simulink model "Quadcopter_LQG_Discrete"  (R2016b)
settings: Solver=ode45  StartTime=0.0  StopTime=33  RelTol=1e-3  EnableMultiTasking=on
undefined symbols (not defined in the file): A, B, C, D, F, kest, Ts, X0
settings Model: Creator=Toshiba  LastModifiedBy=AAstudillo
settings DataIOCC: LimitDataPoints=on  SaveFormat=Array  SignalLoggingSaveFormat=ModelDataLogs
settings OptimizationCC: LifeSpan=inf
settings DebuggingCC: SolverPrmCheckMsg=warning  MultiTaskDSMMsg=warning  MultiTaskCondExecSysMsg=none  SFUnexpectedBacktrackingDiag=warning  SFNoUnconditionalDefaultTransitionDiag=warning  SFExecutionAtInitializationDiag=none
settings HardwareCC: ProdBitPerPointer=32  ProdBitPerSizeT=32  ProdBitPerPtrDiffT=32  ProdLargestAtomicFloat=None  ProdIntDivRoundTo=Undefined  ProdEndianess=Unspecified  ProdWordSize=32  ProdHWDeviceType=32-bit Generic
settings ModelReferenceCC: PropagateSignalLabelsOutOfModel=off
settings GRTTargetCC: TargetLangStandard=C89/C90 (ANSI)  GeneratePreprocessorConditionals=Disable all
settings ConfigComp: CovMetricSettings=dw  CovHtmlReporting=on  CovSaveCumulativeToWorkspaceVar=on  CovSaveSingleToWorkspaceVar=on  CovExternalEMLEnable=off

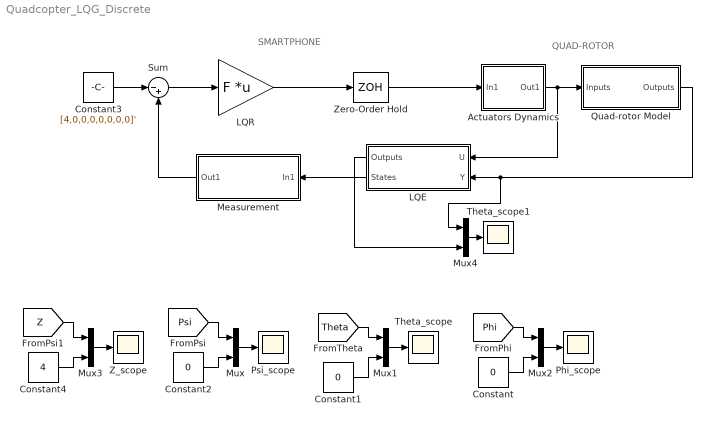
== system Quadcopter_LQG_Discrete ==
  note: QUAD-ROTOR
  note: SMARTPHONE
  Actuators Dynamics : Subsystem
  Constant : Constant  Value=0
  Constant1 : Constant  Value=0
  Constant2 : Constant  Value=0
  Constant3 : Constant  Value=[4,0,0,0,0,0,0,0]'
  Constant4 : Constant  Value=4
  LQE : Subsystem
  LQR : Gain  Gain=F  Multiplication=Matrix(K*u)
  Measurement : Subsystem
  Mux{,1..4} (5 alike) : Mux  Inputs=2
  Phi_scope : Scope
  Psi_scope : Scope
  Quad-rotor Model : Subsystem
  Sum : Sum  Inputs=|-+
  Theta_scope : Scope
  Theta_scope1 : Scope
  Z_scope : Scope
  Zero-Order Hold : ZeroOrderHold  SampleTime=Ts
  wires:
  Constant3/1 -> Sum/1
  Mux/1 -> Psi_scope/1
  Mux1/1 -> Theta_scope/1
  Mux2/1 -> Phi_scope/1
  [Psi] -> Mux/1
  Constant2/1 -> Mux/2
  [Theta] -> Mux1/1
  Constant1/1 -> Mux1/2
  [Phi] -> Mux2/1
  Constant/1 -> Mux2/2
  Actuators Dynamics/1(Out1) -> LQE/1(U), Quad-rotor Model/1(Inputs)
  Sum/1 -> LQR/1
  LQR/1 -> Zero-Order Hold/1
  Zero-Order Hold/1 -> Actuators Dynamics/1(In1)
  Measurement/1(Out1) -> Sum/2
  Mux3/1 -> Z_scope/1
  [Z] -> Mux3/1
  Constant4/1 -> Mux3/2
  LQE/2(States) -> Measurement/1(In1)
  Mux4/1 -> Theta_scope1/1
  Quad-rotor Model/1(Outputs) -> Mux4/1, LQE/2(Y)
  LQE/1(Outputs) -> Mux4/2

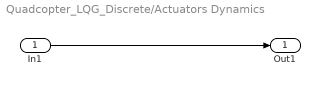
== system Quadcopter_LQG_Discrete/Actuators Dynamics ==
  In1 : Inport
  Out1 : Outport
  wires:
  In1/1 -> Out1/1

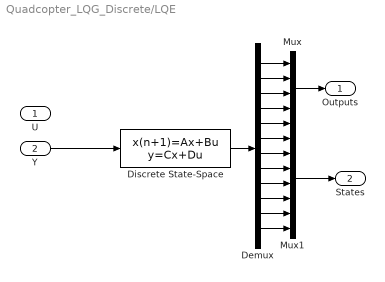
== system Quadcopter_LQG_Discrete/LQE ==
  U : Inport
  Y : Inport  Port=2
  Demux : Demux  Outputs=12
  Discrete State-Space : DiscreteStateSpace  A=kest.A  B=kest.B  C=kest.C  D=kest.D  SampleTime=Ts
  Mux : Mux
  Mux1 : Mux  Inputs=8
  Outputs : Outport
  States : Outport  Port=2
  wires:
  Y/1 -> Discrete State-Space/1
  Discrete State-Space/1 -> Demux/1
  Demux/3 -> Mux/3
  Demux/1 -> Mux/1
  Demux/2 -> Mux/2
  Demux/4 -> Mux/4
  Demux/5 -> Mux1/1
  Demux/6 -> Mux1/2
  Demux/7 -> Mux1/3
  Demux/8 -> Mux1/4
  Demux/9 -> Mux1/5
  Demux/11 -> Mux1/7
  Demux/10 -> Mux1/6
  Demux/12 -> Mux1/8
  Mux/1 -> Outputs/1
  Mux1/1 -> States/1

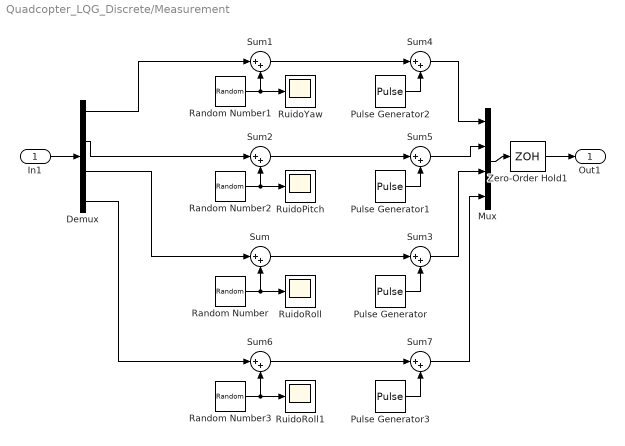
== system Quadcopter_LQG_Discrete/Measurement ==
  In1 : Inport
  Demux : Demux
  Mux : Mux
  Pulse Generator : DiscretePulseGenerator  PulseType=Time based  Amplitude=0.2  Period=10  PulseWidth=5
  Pulse Generator1 : DiscretePulseGenerator  PulseType=Time based  Amplitude=0.2  Period=10  PulseWidth=5
  Pulse Generator2 : DiscretePulseGenerator  PulseType=Time based  Amplitude=0.5  Period=10  PulseWidth=5
  Pulse Generator3 : DiscretePulseGenerator  PulseType=Time based  Amplitude=0.2  Period=10  PulseWidth=5
  Random Number : RandomNumber  Variance=0.01  SampleTime=Ts
  Random Number1 : RandomNumber  Variance=0.3  SampleTime=Ts
  Random Number2 : RandomNumber  Variance=0.01  SampleTime=Ts
  Random Number3 : RandomNumber  Variance=0.01  SampleTime=Ts
  RuidoPitch : Scope
  RuidoRoll : Scope
  RuidoRoll1 : Scope
  RuidoYaw : Scope
  Sum{,1..7} (8 alike) : Sum  Inputs=|++
  Zero-Order Hold1 : ZeroOrderHold  SampleTime=Ts
  Out1 : Outport
  wires:
  Zero-Order Hold1/1 -> Out1/1
  Mux/1 -> Zero-Order Hold1/1
  Random Number/1 -> Sum/2, RuidoRoll/1
  Demux/3 -> Sum/1
  Demux/1 -> Sum1/1
  Random Number2/1 -> RuidoPitch/1, Sum2/2
  Demux/2 -> Sum2/1
  Random Number1/1 -> RuidoYaw/1, Sum1/2
  In1/1 -> Demux/1
  Pulse Generator/1 -> Sum3/2
  Pulse Generator1/1 -> Sum5/2
  Pulse Generator2/1 -> Sum4/2
  Sum2/1 -> Sum5/1
  Sum1/1 -> Sum4/1
  Sum/1 -> Sum3/1
  Sum4/1 -> Mux/1
  Sum5/1 -> Mux/2
  Sum3/1 -> Mux/3
  Random Number3/1 -> Sum6/2, RuidoRoll1/1
  Demux/4 -> Sum6/1
  Pulse Generator3/1 -> Sum7/2
  Sum6/1 -> Sum7/1
  Sum7/1 -> Mux/4

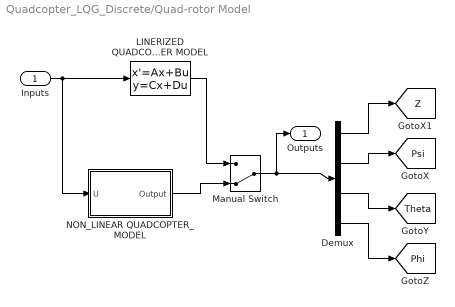
== system Quadcopter_LQG_Discrete/Quad-rotor Model ==
  Inputs : Inport
  Demux : Demux
  LINERIZED QUADCOPTER MODEL : StateSpace  A=A  B=B  C=C  D=D  X0=X0
  Manual Switch : ManualSwitch  CurrentSetting=0
  NON_LINEAR QUADCOPTER_MODEL : Subsystem
  Outputs : Outport
  tag scope: Phi=global, Psi=global, Theta=global, Z=global
  wires:
  Inputs/1 -> LINERIZED QUADCOPTER MODEL/1, NON_LINEAR QUADCOPTER_MODEL/1(U)
  LINERIZED QUADCOPTER MODEL/1 -> Manual Switch/1
  Manual Switch/1 -> Outputs/1, Demux/1
  NON_LINEAR QUADCOPTER_MODEL/1("Output ") -> Manual Switch/2
  Demux/1 -> [Z]
  Demux/2 -> [Psi]
  Demux/3 -> [Theta]
  Demux/4 -> [Phi]

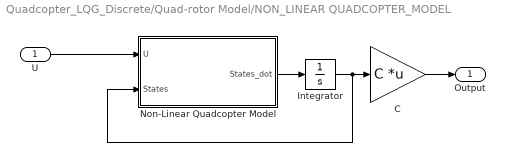
== system Quadcopter_LQG_Discrete/Quad-rotor Model/NON_LINEAR QUADCOPTER_MODEL ==
  U : Inport
  C : Gain  Gain=C  Multiplication=Matrix(K*u)
  Integrator : Integrator  InitialCondition=X0
  Non-Linear Quadcopter Model : MATLAB Function  TreatAsAtomicUnit=on
  "Output " : Outport
  wires:
  Non-Linear Quadcopter Model/1(States_dot) -> Integrator/1
  U/1 -> Non-Linear Quadcopter Model/1(U)
  Integrator/1 -> C/1, Non-Linear Quadcopter Model/2(States)
  C/1 -> "Output "/1

== matlab function Quadcopter_LQG_Discrete/Quad-rotor Model/NON_LINEAR QUADCOPTER_MODEL/Non-Linear Quadcopter Model ==
  data: U input; States input; States_dot output
function States_dot  = fcn(U, States)
   
    % Gravity constant
              g = 9.807;

              m = 1.5680;
              Ixx = 0.0135;
              Iyy = 0.0124;
              Izz = 0.0336;

    %Inputs = U, States
    %Outputs = States_dot  
    %States: Z dZ Psi dPsi Theta dTheta Phi dPhi
    %        1  2  3  4      5      6     7   8
    
    U1 = U(1);
    U2 = U(2);
    U3 = U(3);
    U4 = U(4);
    
    dZ = States(2);
    ddZ = -g*cos(States(5))*cos(States(7)) + (cos(States(5))*cos(States(7)))*(U1+m*g)/m;
    dPsi = States(4);
    ddPsi = (((Ixx-Iyy)/Izz)*States(8)*States(6)) + (U2/Izz);
    dTheta = States(6);
    ddTheta = (((Izz-Ixx)/Iyy)*States(8)*States(4)) + (U3/Iyy);
    dPhi = States(8);
    ddPhi = (((Iyy-Izz)/Ixx)*States(6)*States(4)) + (U4/Ixx);

    States_dot = [dZ, ddZ, dPsi, ddPsi, dTheta, ddTheta, dPhi, ddPhi]';
